simulink model "Module5"  (R2021b)
settings: Solver=VariableStepAuto  StartTime=0.0  StopTime=40.0  RelTol=1e-3
libraries: simulink x3
settings Model: Creator=Lenovo  LastModifiedBy=Lenovo

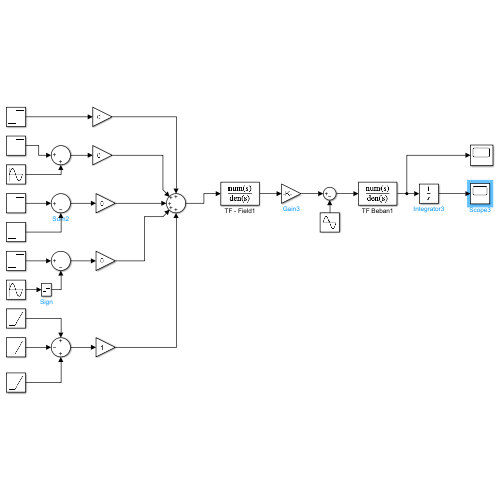
[thumbnail: Simulink's stored preview of the top-level diagram]
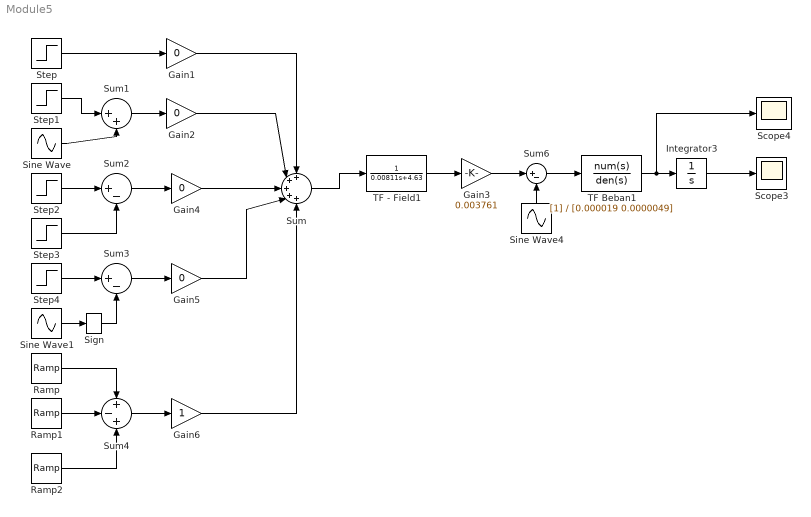
== system Module5 ==
  Gain{1..2,4..5} (4 alike) : Gain  Gain=0
  Gain3 : Gain  Gain=0.003761
  Gain6 : Gain
  Integrator3 : Integrator
  Ramp : simulink/Sources/Ramp  slope=1  start=0  InitialOutput=0
  Ramp1 : simulink/Sources/Ramp  slope=2  start=5  InitialOutput=0
  Ramp2 : simulink/Sources/Ramp  slope=10  start=10  InitialOutput=0
  Scope3 : Scope
  Scope4 : Scope
  Sign : Signum
  Sine Wave : Sin  Amplitude=0.1  Frequency=2*pi  SampleTime=0
  Sine Wave1 : Sin  Frequency=2*pi  SampleTime=0
  Sine Wave4 : Sin  Amplitude=0.0005  Frequency=2*pi  SampleTime=0
  Step{,1..2,4} (4 alike) : Step  Time=0  SampleTime=0
  Step3 : Step  Time=5  SampleTime=0
  Sum : Sum  Inputs=+++++
  Sum1 : Sum  Inputs=|++
  Sum2 : Sum  Inputs=|+-
  Sum3 : Sum  Inputs=|+-
  Sum4 : Sum  Inputs=+-+
  Sum6 : Sum  Inputs=|+-
  TF - Field1 : TransferFcn  Denominator=[0.00811 4.63]
  TF Beban1 : TransferFcn  Denominator=[0.000019 0.0000049]
  wires:
  Sum6/1 -> TF Beban1/1
  TF Beban1/1 -> Scope4/1, Integrator3/1
  Gain3/1 -> Sum6/1
  TF - Field1/1 -> Gain3/1
  Sine Wave4/1 -> Sum6/2
  Integrator3/1 -> Scope3/1
  Sum/1 -> TF - Field1/1
  Gain1/1 -> Sum/1
  Gain2/1 -> Sum/2
  Gain4/1 -> Sum/3
  Gain5/1 -> Sum/4
  Gain6/1 -> Sum/5
  Step/1 -> Gain1/1
  Step1/1 -> Sum1/1
  Sine Wave/1 -> Sum1/2
  Sum1/1 -> Gain2/1
  Sum2/1 -> Gain4/1
  Step2/1 -> Sum2/1
  Step3/1 -> Sum2/2
  Sum3/1 -> Gain5/1
  Step4/1 -> Sum3/1
  Sine Wave1/1 -> Sign/1
  Sign/1 -> Sum3/2
  Sum4/1 -> Gain6/1
  Ramp/1 -> Sum4/1
  Ramp1/1 -> Sum4/2
  Ramp2/1 -> Sum4/3
